simulink model "test_ROS"  (R2019b)
settings: Solver=VariableStepAuto  StartTime=0.0  StopTime=inf  RelTol=1e-3
libraries: robotlib x2
settings Model: Creator=jiyo  LastModifiedBy=jiyo

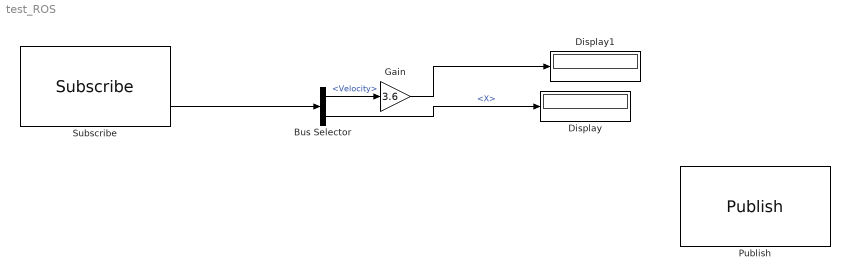
== system test_ROS ==
  Bus Selector : BusSelector  OutputSignals=Velocity,Acceleration.Linear.X
  Display : Display
  Display1 : Display
  Gain : Gain  Gain=3.6
  Publish : robotlib/Publish  topicSource=Select from ROS network  topic=/carla/ego_vehicle/vehicle_control_cmd_manual  messageType=carla_msgs/CarlaEgoVehicleControl  messageQueueLength=1
      settings: SourceProductName=ROS Toolbox
  Subscribe : robotlib/Subscribe  topicSource=Select from ROS network  topic=/carla/ego_vehicle/vehicle_status  messageType=carla_msgs/CarlaEgoVehicleStatus  sampleTime=-1  messageQueueLength=1
      settings: SourceProductName=ROS Toolbox
  wires:
  Subscribe/2 -> Bus Selector/1
  Bus Selector/2 -> Display/1  "<X>"
  Bus Selector/1 -> Gain/1  "<Velocity>"
  Gain/1 -> Display1/1
